simulink model "ReemcROStestlink"  (R2015a)
settings: Solver=ode45  StartTime=0.0  StopTime=inf  RelTol=1e-3
model workspace (MAT data in the model file):
  SL_ROS_VariableLengthArrays_MaxSizes.CommonInfo.ArrayTruncateAction = 'EmitWarning'
  SL_ROS_VariableLengthArrays_MaxSizes.MsgTypeMap = containers.Map
  SL_ROS_VariableLengthArrays_MaxSizes.MsgTypeMap.serialization.keys = {'gazebo_msgs/LinkStates'}
  SL_ROS_VariableLengthArrays_MaxSizes.MsgTypeMap.serialization.values{1}(1).PropertyName = 'Pose'
  SL_ROS_VariableLengthArrays_MaxSizes.MsgTypeMap.serialization.values{1}(1).DataType = 'geometry_msgs/Pose'
  SL_ROS_VariableLengthArrays_MaxSizes.MsgTypeMap.serialization.values{1}(1).MaxLength = 60
  SL_ROS_VariableLengthArrays_MaxSizes.MsgTypeMap.serialization.values{1}(2).PropertyName = 'Twist'
  SL_ROS_VariableLengthArrays_MaxSizes.MsgTypeMap.serialization.values{1}(2).DataType = 'geometry_msgs/Twist'
  SL_ROS_VariableLengthArrays_MaxSizes.MsgTypeMap.serialization.values{1}(2).MaxLength = 60
  SL_ROS_VariableLengthArrays_MaxSizes.MsgTypeMap.serialization.uniformity = 0
  SL_ROS_VariableLengthArrays_MaxSizes.MsgTypeMap.serialization.keyType = 'char'
  SL_ROS_VariableLengthArrays_MaxSizes.MsgTypeMap.serialization.valueType = 'any'
values from neighbouring files (symbols this model uses):
  left_ft = struct('force',0,'torqueX',0,'torqueY',0)    [Feedback.m]
  right_ft = struct('force',0,'torqueX',0,'torqueY',0)    [Feedback.m]
libraries: robotlib x13
settings Model: Creator=jifeixu  LastModifiedBy=jifeixu
settings OptimizationCC: BlockReduction=off  BufferReuse=off
settings DebuggingCC: AlgebraicLoopMsg=none  UnconnectedInputMsg=none  UnconnectedOutputMsg=none  UnconnectedLineMsg=none

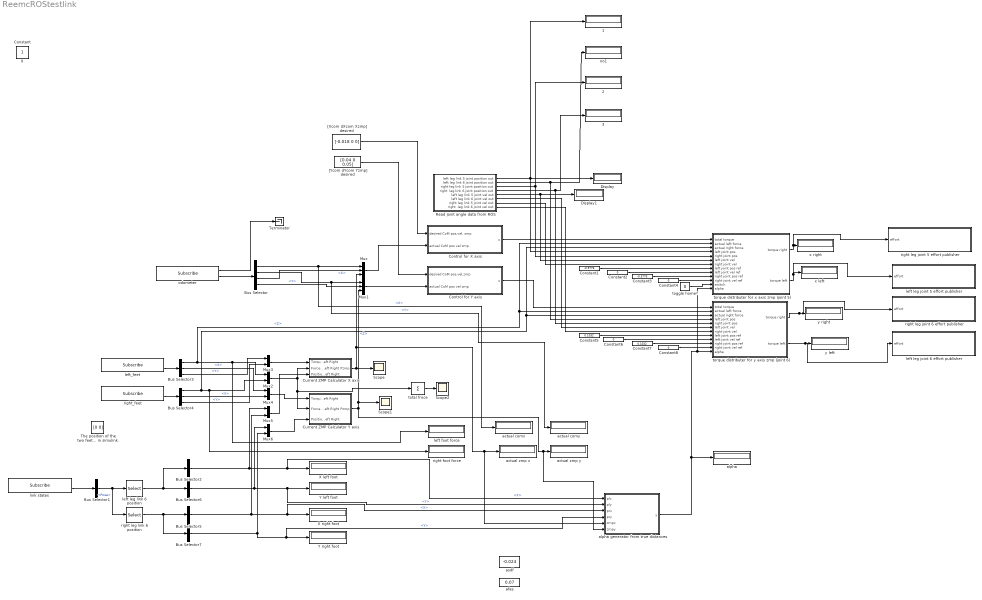
== system ReemcROStestlink ==
  1 : Display
  2 : Display
  3 : Display
  Bus Selector : BusSelector  OutputSignals=Pose.Pose.Position.X,Pose.Pose.Position.Y,Twist.Twist.Linear.X,Twist.Twist.Linear.Y
  Bus Selector1 : BusSelector  OutputSignals=Pose
  Bus Selector2 : BusSelector  OutputSignals=Position.X
  Bus Selector3 : BusSelector  OutputSignals=Wrench.Force.Z,Wrench.Torque.X,Wrench.Torque.Y
  Bus Selector4 : BusSelector  OutputSignals=Wrench.Force.Z,Wrench.Torque.X,Wrench.Torque.Y
  Bus Selector5 : BusSelector  OutputSignals=Position.X
  Bus Selector6 : BusSelector  OutputSignals=Position.Y
  Bus Selector7 : BusSelector  OutputSignals=Position.Y
  Constant1 : Constant  Value=-0.5776
  Constant{2,4,6,8} (4 alike) : Constant  Value=0
  Constant3 : Constant  Value=-0.5776
  Constant5 : Constant  Value=0.1032
  Constant7 : Constant  Value=0.1032
  Control for X axis : Subsystem
  Control for Y axis : Subsystem
  Current ZMP Calculator X axis : Subsystem
  Current ZMP Calculator Y axis : Subsystem
  Display : Display
  Display1 : Display
  Mux : Mux  Inputs=3
  Mux1 : Mux  Inputs=3
  Mux{2..6} (5 alike) : Mux  Inputs=2
  Read joint angle data from ROS : Subsystem
  Scope : Scope
      settings: YMin=-0.08  YMax=0.14
  Scope1 : Scope
      settings: YMin=-0.225  YMax=0.05
  Scope2 : Scope
      settings: YMin=-100  YMax=1700  SaveName=ScopeData2
  Terminator : Terminator
  The position of the two feet that should have come from the link state subscriber but currently does not work in simulink. : Constant  Value=[0 0]
  X left foot : Display
  X right foot : Display
  Y left foot : Display
  Y right foot : Display
  "[Xcom dXcom Xzmp] desired" : Constant  Value=[-0.018 0 0]  VectorParams1D=off
  "[Ycom dYcom Yzmp] desired" : Constant  Value=[0.04 0 0.05]  VectorParams1D=off
  actual comx : Display
  actual comy : Display
  actual zmp x : Display
  actual zmp y : Display
  afas : Constant  Value=0.07
  alpha : Display
  alpha generator from true distances : MATLAB Function  TreatAsAtomicUnit=on
  asdf : Constant  Value=-0.024
  left foot force : Display
  left leg joint 5 effort publisher : Subsystem
  left leg joint 6 effort publisher : Subsystem
  left leg link 6 position : Selector  InputPortWidth=60  Indices=8  OutputSizes=2
  left_feet : robotlib/Subscribe  SourceLibraryInfo=This block requires Robotics System Toolbox  topicSource=Select from ROS network  topic=/left_ft  messageType=geometry_msgs/WrenchStamped  sampleTime=-1  messageQueueLength=1
  link states : robotlib/Subscribe  SourceLibraryInfo=This block requires Robotics System Toolbox  topicSource=Select from ROS network  topic=/gazebo/link_states  messageType=gazebo_msgs/LinkStates  sampleTime=-1  messageQueueLength=1
  no1 : Display
  odometer : robotlib/Subscribe  SourceLibraryInfo=This block requires Robotics System Toolbox  topicSource=Select from ROS network  topic=/ground_truth_odom  messageType=nav_msgs/Odometry  sampleTime=-1  messageQueueLength=1
  right foot force : Display
  right leg joint 5 effort publisher : Subsystem
  right leg joint 6 effort publisher : Subsystem
  right leg link 6 position : Selector  InputPortWidth=60  Indices=14  OutputSizes=2
  right_feet : robotlib/Subscribe  SourceLibraryInfo=This block requires Robotics System Toolbox  topicSource=Select from ROS network  topic=/right_ft  messageType=geometry_msgs/WrenchStamped  sampleTime=-1  messageQueueLength=1
  toggle home? : Constant  Value=0
  torque distributer for x axis zmp (joint 5) : Subsystem
  torque distributer for y axis zmp (joint 6) : Subsystem
  total froce : Sum  Inputs=+
  x left : Display
  x right : Display
  y left : Display
  y right : Display
  0 : Constant  IOType=siggen
  Constant : Constant  IOType=siggen
  wires:
  odometer/2 -> Bus Selector/1
  odometer/1 -> Terminator/1
  left_feet/2 -> Bus Selector3/1
  right_feet/2 -> Bus Selector4/1
  Bus Selector/1 -> actual comx/1, Mux/1  "<X>"
  Bus Selector/3 -> Mux/2  "<X>"
  Bus Selector/2 -> actual comy/1, Mux1/1  "<Y>"
  Bus Selector/4 -> Mux1/2  "<Y>"
  Current ZMP Calculator X axis/1(Pzmp) -> Scope/1, alpha generator from true distances/5(zmpx), actual zmp x/1, Mux/3
  Current ZMP Calculator Y axis/1(Pzmp) -> Mux1/3, Scope1/1, alpha generator from true distances/6(zmpy), actual zmp y/1
  "[Xcom dXcom Xzmp] desired"/1 -> Control for X axis/1("desired CoM pos,vel, zmp")
  Mux/1 -> Control for X axis/2("actual CoM pos vel zmp ")
  Mux2/1 -> total froce/1, Current ZMP Calculator Y axis/2(Force Left Right), Current ZMP Calculator X axis/2(Force Left Right)
  Bus Selector3/1 -> torque distributer for y axis zmp (joint 6)/2(actual left force), torque distributer for x axis zmp (joint 5)/2(actual left force), left foot force/1, Mux2/1  "<Z>"
  Bus Selector4/1 -> torque distributer for y axis zmp (joint 6)/3(actual right force), torque distributer for x axis zmp (joint 5)/3(actual right force), right foot force/1, Mux2/2  "<Z>"
  Mux3/1 -> Current ZMP Calculator X axis/1(Torque Left Right)
  Mux4/1 -> Current ZMP Calculator Y axis/1(Torque Left Right)
  Bus Selector3/3 -> Mux3/1  "<Y>"
  Bus Selector4/3 -> Mux3/2  "<Y>"
  Bus Selector3/2 -> Mux4/1  "<X>"
  Bus Selector4/2 -> Mux4/2  "<X>"
  Mux1/1 -> Control for Y axis/2("actual CoM pos vel zmp ")
  "[Ycom dYcom Yzmp] desired"/1 -> Control for Y axis/1(desired CoM pos,vel,zmp)
  link states/2 -> Bus Selector1/1
  Bus Selector1/1 -> right leg link 6 position/1, left leg link 6 position/1  "<Pose>"
  Bus Selector2/1 -> Mux5/1, alpha generator from true distances/1(plx), X left foot/1  "<X>"
  Control for X axis/1(u) -> torque distributer for x axis zmp (joint 5)/1(total torque)
  left leg link 6 position/1 -> Bus Selector2/1, Bus Selector6/1
  Bus Selector5/1 -> Mux5/2, alpha generator from true distances/3(prx), X right foot/1  "<X>"
  right leg link 6 position/1 -> Bus Selector7/1, Bus Selector5/1
  Bus Selector6/1 -> Mux6/1, alpha generator from true distances/2(ply), Y left foot/1  "<Y>"
  Bus Selector7/1 -> alpha generator from true distances/4(pry), Y right foot/1, Mux6/2  "<Y>"
  Mux5/1 -> Current ZMP Calculator X axis/3(Position Left Right)
  Mux6/1 -> Current ZMP Calculator Y axis/3(Position Left Right)
  total froce/1 -> Scope2/1
  Read joint angle data from ROS/1(left leg link 5 joint position out) -> Display/1, 1/1, torque distributer for x axis zmp (joint 5)/4(left joint pos)
  Read joint angle data from ROS/3(right leg link 5 joint position out) -> torque distributer for x axis zmp (joint 5)/5(right joint pos), 2/1
  Read joint angle data from ROS/2(left leg link 6 joint position out) -> torque distributer for y axis zmp (joint 6)/4(left joint pos), no1/1
  Read joint angle data from ROS/4(right  leg link 6 joint position out) -> torque distributer for y axis zmp (joint 6)/5(right joint pos), 3/1
  Read joint angle data from ROS/5(left leg link 5 joint vel out) -> Display1/1, torque distributer for x axis zmp (joint 5)/6(left joint vel)
  Read joint angle data from ROS/7(right leg link 5 joint vel out) -> torque distributer for x axis zmp (joint 5)/7(right joint vel)
  torque distributer for x axis zmp (joint 5)/1(torque right) -> right leg joint 5 effort publisher/1(effort), x right/1
  torque distributer for x axis zmp (joint 5)/2(torque left) -> x left/1, left leg joint 5 effort publisher/1(effort)
  Read joint angle data from ROS/6(left leg link 6 joint vel out) -> torque distributer for y axis zmp (joint 6)/6(left joint vel)
  Read joint angle data from ROS/8(right  leg link 6 joint vel out) -> torque distributer for y axis zmp (joint 6)/7(right joint vel)
  torque distributer for y axis zmp (joint 6)/1(torque right) -> right leg joint 6 effort publisher/1(effort), y right/1
  Control for Y axis/1(u) -> torque distributer for y axis zmp (joint 6)/1(total torque)
  Constant1/1 -> torque distributer for x axis zmp (joint 5)/8(left joint pos ref)
  Constant2/1 -> torque distributer for x axis zmp (joint 5)/9(left joint vel ref)
  Constant3/1 -> torque distributer for x axis zmp (joint 5)/10(right joint pos ref)
  Constant4/1 -> torque distributer for x axis zmp (joint 5)/11(right joint vel ref)
  Constant5/1 -> torque distributer for y axis zmp (joint 6)/8(left joint pos ref)
  Constant6/1 -> torque distributer for y axis zmp (joint 6)/9(left joint vel ref)
  Constant7/1 -> torque distributer for y axis zmp (joint 6)/10(right joint pos ref)
  Constant8/1 -> torque distributer for y axis zmp (joint 6)/11(right joint vel ref)
  torque distributer for y axis zmp (joint 6)/2(torque left) -> left leg joint 6 effort publisher/1(effort), y left/1
  toggle home?/1 -> torque distributer for x axis zmp (joint 5)/12(switch)
  alpha generator from true distances/1(y) -> alpha/1, torque distributer for x axis zmp (joint 5)/13(alpha), torque distributer for y axis zmp (joint 6)/12(alpha)

== system ReemcROStestlink/Control for X axis ==
  "desired CoM pos,vel, zmp" : Inport
  "actual CoM pos vel zmp " : Inport  Port=2
  Add : Sum
  Demux : Demux  Outputs=3
  K gains : Constant  Value="[ -3235   -150    20.5]"  VectorParams1D=off
  Permute Dimensions : PermuteDimensions
  Product : Product  Multiplication=Matrix(*)
  Subtract : Sum  Inputs=+-
  u : Outport
  wires:
  "desired CoM pos,vel, zmp"/1 -> Demux/1, Subtract/1
  K gains/1 -> Product/1
  Subtract/1 -> Permute Dimensions/1
  "actual CoM pos vel zmp "/1 -> Subtract/2
  Product/1 -> Add/2
  Add/1 -> u/1
  Demux/3 -> Add/1
  Permute Dimensions/1 -> Product/2

== system ReemcROStestlink/Control for Y axis ==
  desired CoM pos,vel,zmp : Inport
  "actual CoM pos vel zmp " : Inport  Port=2
  Add : Sum
  Demux : Demux  Outputs=3
  K gains : Constant  Value="[ -3235   -150    20.5]"  VectorParams1D=off
  Permute Dimensions : PermuteDimensions
  Product : Product  Multiplication=Matrix(*)
  Subtract : Sum  Inputs=+-
  u : Outport
  wires:
  K gains/1 -> Product/1
  "actual CoM pos vel zmp "/1 -> Subtract/2
  Product/1 -> Add/2
  Add/1 -> u/1
  Permute Dimensions/1 -> Product/2
  Subtract/1 -> Permute Dimensions/1
  desired CoM pos,vel,zmp/1 -> Demux/1, Subtract/1
  Demux/3 -> Add/1

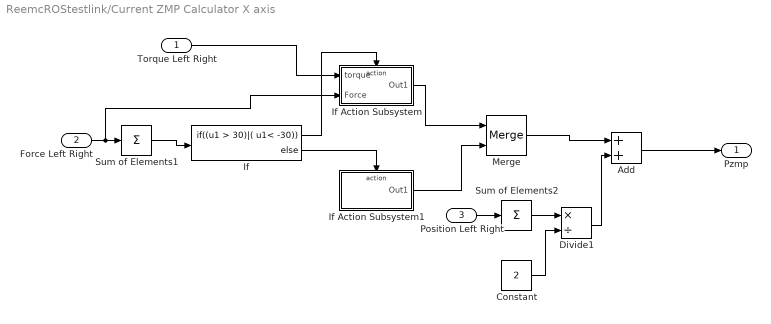
== system ReemcROStestlink/Current ZMP Calculator X axis ==
  Torque Left Right : Inport
  Force Left Right : Inport  Port=2
  Position Left Right : Inport  Port=3
  Add : Sum
  Constant : Constant  Value=2
  Divide1 : Product  Inputs=*/
  If : If  IfExpression=(u1 > 30)|( u1< -30)
  If Action Subsystem : Subsystem  TreatAsAtomicUnit=on
  If Action Subsystem1 : Subsystem  TreatAsAtomicUnit=on
  Merge : Merge
  Sum of Elements1 : Sum  Inputs=+
  Sum of Elements2 : Sum  Inputs=+
  Pzmp : Outport
  wires:
  Force Left Right/1 -> If Action Subsystem/2(Force), Sum of Elements1/1
  Sum of Elements1/1 -> If/1
  If Action Subsystem1/1(Out1) -> Merge/2
  Merge/1 -> Add/1
  Add/1 -> Pzmp/1
  Position Left Right/1 -> Sum of Elements2/1
  Sum of Elements2/1 -> Divide1/1
  Constant/1 -> Divide1/2
  Divide1/1 -> Add/2
  Torque Left Right/1 -> If Action Subsystem/1(torque)
  If Action Subsystem/1(Out1) -> Merge/1
  If/1 -> If Action Subsystem/Action
  If/2 -> If Action Subsystem1/Action

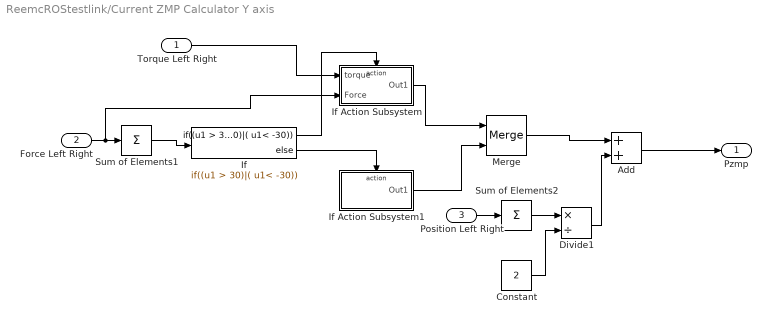
== system ReemcROStestlink/Current ZMP Calculator Y axis ==
  Torque Left Right : Inport
  Force Left Right : Inport  Port=2
  Position Left Right : Inport  Port=3
  Add : Sum
  Constant : Constant  Value=2
  Divide1 : Product  Inputs=*/
  If : If  IfExpression=(u1 > 30)|( u1< -30)
  If Action Subsystem : Subsystem  TreatAsAtomicUnit=on
  If Action Subsystem1 : Subsystem  TreatAsAtomicUnit=on
  Merge : Merge
  Sum of Elements1 : Sum  Inputs=+
  Sum of Elements2 : Sum  Inputs=+
  Pzmp : Outport
  wires:
  Force Left Right/1 -> If Action Subsystem/2(Force), Sum of Elements1/1
  Sum of Elements1/1 -> If/1
  If Action Subsystem1/1(Out1) -> Merge/2
  Merge/1 -> Add/1
  Add/1 -> Pzmp/1
  Position Left Right/1 -> Sum of Elements2/1
  Sum of Elements2/1 -> Divide1/1
  Constant/1 -> Divide1/2
  Divide1/1 -> Add/2
  Torque Left Right/1 -> If Action Subsystem/1(torque)
  If Action Subsystem/1(Out1) -> Merge/1
  If/1 -> If Action Subsystem/Action
  If/2 -> If Action Subsystem1/Action

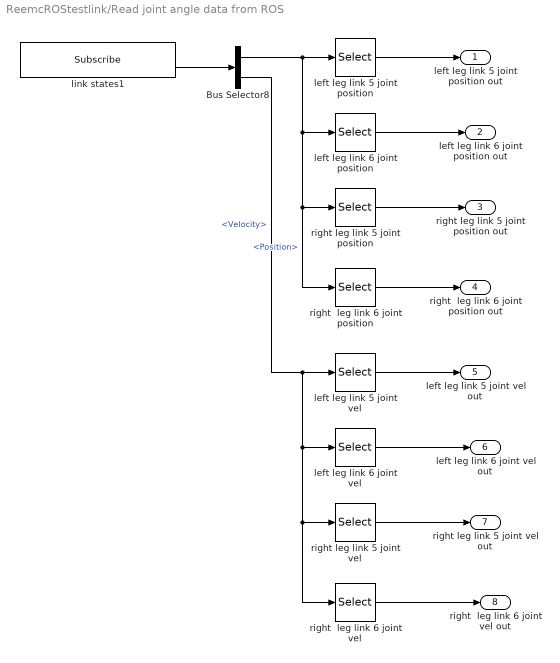
== system ReemcROStestlink/Read joint angle data from ROS ==
  Bus Selector8 : BusSelector  OutputSignals=Position,Velocity
  left leg link 5 joint position : Selector  InputPortWidth=128  Indices=39  OutputSizes=2
  left leg link 5 joint vel : Selector  InputPortWidth=128  Indices=39  OutputSizes=2
  left leg link 6 joint position : Selector  InputPortWidth=128  Indices=40  OutputSizes=2
  left leg link 6 joint vel : Selector  InputPortWidth=128  Indices=40  OutputSizes=2
  link states1 : robotlib/Subscribe  SourceLibraryInfo=This block requires Robotics System Toolbox  topicSource=Select from ROS network  topic=/joint_states  messageType=sensor_msgs/JointState  sampleTime=-1  messageQueueLength=1
  right  leg link 6 joint position : Selector  InputPortWidth=128  Indices=46  OutputSizes=2
  right  leg link 6 joint vel : Selector  InputPortWidth=128  Indices=46  OutputSizes=2
  right leg link 5 joint position : Selector  InputPortWidth=128  Indices=45  OutputSizes=2
  right leg link 5 joint vel : Selector  InputPortWidth=128  Indices=45  OutputSizes=2
  left leg link 5 joint position out : Outport
  left leg link 6 joint position out : Outport  Port=2
  right leg link 5 joint position out : Outport  Port=3
  right  leg link 6 joint position out : Outport  Port=4
  left leg link 5 joint vel out : Outport  Port=5
  left leg link 6 joint vel out : Outport  Port=6
  right leg link 5 joint vel out : Outport  Port=7
  right  leg link 6 joint vel out : Outport  Port=8
  wires:
  Bus Selector8/1 -> left leg link 6 joint position/1, right  leg link 6 joint position/1, right leg link 5 joint position/1, left leg link 5 joint position/1  "<Position>"
  left leg link 5 joint position/1 -> left leg link 5 joint position out/1
  left leg link 6 joint position/1 -> left leg link 6 joint position out/1
  link states1/2 -> Bus Selector8/1
  right leg link 5 joint position/1 -> right leg link 5 joint position out/1
  right  leg link 6 joint position/1 -> right  leg link 6 joint position out/1
  Bus Selector8/2 -> left leg link 6 joint vel/1, right  leg link 6 joint vel/1, right leg link 5 joint vel/1, left leg link 5 joint vel/1  "<Velocity>"
  left leg link 5 joint vel/1 -> left leg link 5 joint vel out/1
  left leg link 6 joint vel/1 -> left leg link 6 joint vel out/1
  right leg link 5 joint vel/1 -> right leg link 5 joint vel out/1
  right  leg link 6 joint vel/1 -> right  leg link 6 joint vel out/1

== system ReemcROStestlink/left leg joint 5 effort publisher ==
  effort : Inport
  Blank Message : robotlib/Blank Message  SourceLibraryInfo=This block requires Robotics System Toolbox  messageType=std_msgs/Float64  SampleTime=inf
  Bus Assignment : BusAssignment  AssignedSignals=Data
  Publish : robotlib/Publish  SourceLibraryInfo=This block requires Robotics System Toolbox  topicSource=Select from ROS network  topic=/left_leg_effort_controller2/command  messageType=std_msgs/Float64  messageQueueLength=1
  wires:
  effort/1 -> Bus Assignment/2
  Bus Assignment/1 -> Publish/1
  Blank Message/1 -> Bus Assignment/1

== system ReemcROStestlink/left leg joint 6 effort publisher ==
  effort : Inport
  Blank Message : robotlib/Blank Message  SourceLibraryInfo=This block requires Robotics System Toolbox  messageType=std_msgs/Float64  SampleTime=inf
  Bus Assignment : BusAssignment  AssignedSignals=Data
  Publish : robotlib/Publish  SourceLibraryInfo=This block requires Robotics System Toolbox  topicSource=Select from ROS network  topic=/left_leg_effort_controller3/command  messageType=std_msgs/Float64  messageQueueLength=1
  wires:
  effort/1 -> Bus Assignment/2
  Bus Assignment/1 -> Publish/1
  Blank Message/1 -> Bus Assignment/1

== system ReemcROStestlink/right leg joint 5 effort publisher ==
  effort : Inport
  Blank Message : robotlib/Blank Message  SourceLibraryInfo=This block requires Robotics System Toolbox  messageType=std_msgs/Float64  SampleTime=inf
  Bus Assignment : BusAssignment  AssignedSignals=Data
  Publish2 : robotlib/Publish  SourceLibraryInfo=This block requires Robotics System Toolbox  topicSource=Select from ROS network  topic=/right_leg_effort_controller2/command  messageType=std_msgs/Float64  messageQueueLength=1
  wires:
  effort/1 -> Bus Assignment/2
  Bus Assignment/1 -> Publish2/1
  Blank Message/1 -> Bus Assignment/1

== system ReemcROStestlink/right leg joint 6 effort publisher ==
  effort : Inport
  Blank Message : robotlib/Blank Message  SourceLibraryInfo=This block requires Robotics System Toolbox  messageType=std_msgs/Float64  SampleTime=inf
  Bus Assignment : BusAssignment  AssignedSignals=Data
  Publish2 : robotlib/Publish  SourceLibraryInfo=This block requires Robotics System Toolbox  topicSource=Select from ROS network  topic=/right_leg_effort_controller3/command  messageType=std_msgs/Float64  messageQueueLength=1
  wires:
  effort/1 -> Bus Assignment/2
  Bus Assignment/1 -> Publish2/1
  Blank Message/1 -> Bus Assignment/1

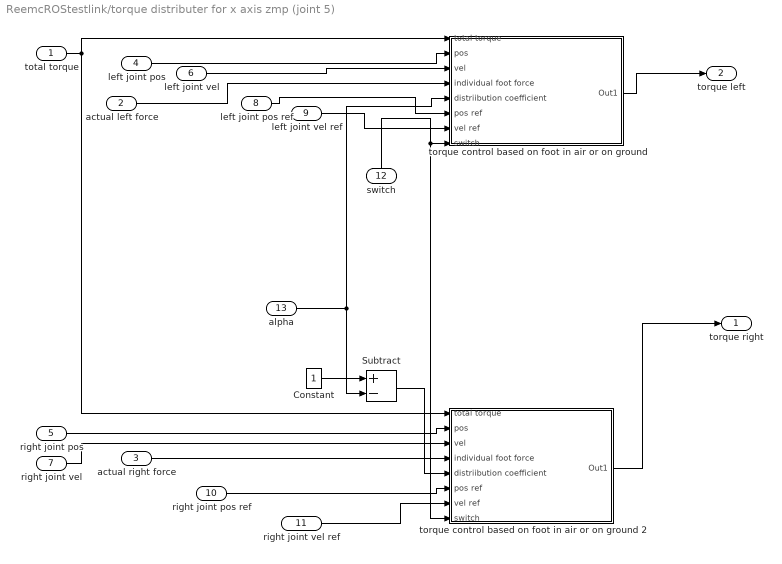
== system ReemcROStestlink/torque distributer for x axis zmp (joint 5) ==
  total torque : Inport
  actual left force : Inport  Port=2
  actual right force : Inport  Port=3
  left joint pos : Inport  Port=4
  right joint pos : Inport  Port=5
  left joint vel : Inport  Port=6
  right joint vel : Inport  Port=7
  left joint pos ref : Inport  Port=8
  left joint vel ref : Inport  Port=9
  right joint pos ref : Inport  Port=10
  right joint vel ref : Inport  Port=11
  switch : Inport  Port=12
  alpha : Inport  Port=13
  Constant : Constant
  Subtract : Sum  Inputs=+-
  torque control based on foot in air or on ground : Subsystem
  torque control based on foot in air or on ground 2 : Subsystem
  torque right : Outport
  torque left : Outport  Port=2
  wires:
  total torque/1 -> torque control based on foot in air or on ground 2/1(total torque), torque control based on foot in air or on ground/1(total torque)
  left joint pos/1 -> torque control based on foot in air or on ground/2(pos)
  left joint vel/1 -> torque control based on foot in air or on ground/3(vel)
  alpha/1 -> Subtract/2, torque control based on foot in air or on ground/5(distriibution coefficient)
  torque control based on foot in air or on ground/1(Out1) -> torque left/1
  right joint pos/1 -> torque control based on foot in air or on ground 2/2(pos)
  right joint vel/1 -> torque control based on foot in air or on ground 2/3(vel)
  Constant/1 -> Subtract/1
  Subtract/1 -> torque control based on foot in air or on ground 2/5(distriibution coefficient)
  torque control based on foot in air or on ground 2/1(Out1) -> torque right/1
  left joint pos ref/1 -> torque control based on foot in air or on ground/6(pos ref)
  left joint vel ref/1 -> torque control based on foot in air or on ground/7(vel ref)
  right joint pos ref/1 -> torque control based on foot in air or on ground 2/6(pos ref)
  right joint vel ref/1 -> torque control based on foot in air or on ground 2/7(vel ref)
  switch/1 -> torque control based on foot in air or on ground 2/8(switch), torque control based on foot in air or on ground/8(switch)
  actual right force/1 -> torque control based on foot in air or on ground 2/4(individual foot force)
  actual left force/1 -> torque control based on foot in air or on ground/4(individual foot force)

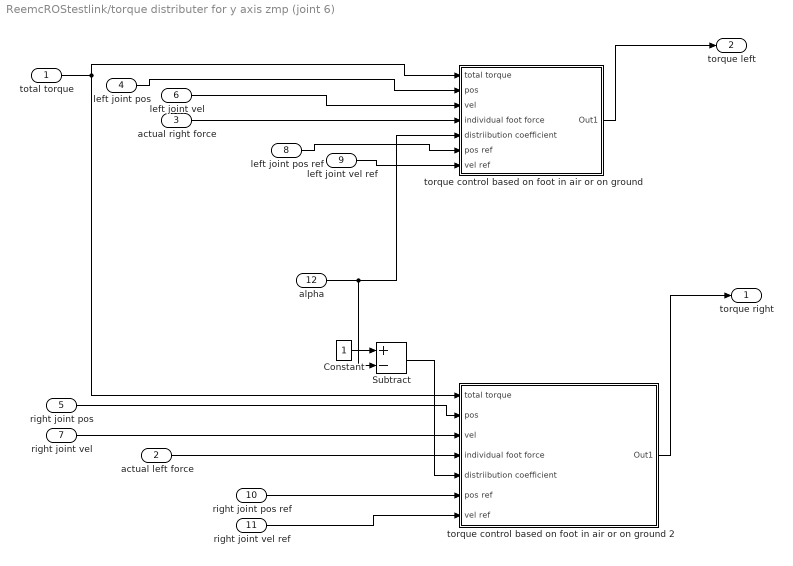
== system ReemcROStestlink/torque distributer for y axis zmp (joint 6) ==
  total torque : Inport
  actual left force : Inport  Port=2
  actual right force : Inport  Port=3
  left joint pos : Inport  Port=4
  right joint pos : Inport  Port=5
  left joint vel : Inport  Port=6
  right joint vel : Inport  Port=7
  left joint pos ref : Inport  Port=8
  left joint vel ref : Inport  Port=9
  right joint pos ref : Inport  Port=10
  right joint vel ref : Inport  Port=11
  alpha : Inport  Port=12
  Constant : Constant
  Subtract : Sum  Inputs=+-
  torque control based on foot in air or on ground : Subsystem
  torque control based on foot in air or on ground 2 : Subsystem
  torque right : Outport
  torque left : Outport  Port=2
  wires:
  actual left force/1 -> torque control based on foot in air or on ground 2/4(individual foot force)
  actual right force/1 -> torque control based on foot in air or on ground/4(individual foot force)
  total torque/1 -> torque control based on foot in air or on ground/1(total torque), torque control based on foot in air or on ground 2/1(total torque)
  left joint pos/1 -> torque control based on foot in air or on ground/2(pos)
  left joint vel/1 -> torque control based on foot in air or on ground/3(vel)
  alpha/1 -> torque control based on foot in air or on ground/5(distriibution coefficient), Subtract/2
  torque control based on foot in air or on ground/1(Out1) -> torque left/1
  right joint pos/1 -> torque control based on foot in air or on ground 2/2(pos)
  right joint vel/1 -> torque control based on foot in air or on ground 2/3(vel)
  Constant/1 -> Subtract/1
  Subtract/1 -> torque control based on foot in air or on ground 2/5(distriibution coefficient)
  torque control based on foot in air or on ground 2/1(Out1) -> torque right/1
  left joint pos ref/1 -> torque control based on foot in air or on ground/6(pos ref)
  left joint vel ref/1 -> torque control based on foot in air or on ground/7(vel ref)
  right joint vel ref/1 -> torque control based on foot in air or on ground 2/7(vel ref)
  right joint pos ref/1 -> torque control based on foot in air or on ground 2/6(pos ref)

== system ReemcROStestlink/Current ZMP Calculator X axis/If Action Subsystem ==
  torque : Inport
  Force : Inport  Port=2
  Action Port : ActionPort  ActionType=then
  Divide : Product  Inputs=*/
  Gain : Gain  Gain=-1
  Sum of Elements : Sum  Inputs=+
  Sum of Elements1 : Sum  Inputs=+
  Out1 : Outport
  wires:
  Divide/1 -> Out1/1
  Gain/1 -> Divide/1
  torque/1 -> Sum of Elements/1
  Sum of Elements/1 -> Gain/1
  Force/1 -> Sum of Elements1/1
  Sum of Elements1/1 -> Divide/2

== system ReemcROStestlink/Current ZMP Calculator X axis/If Action Subsystem1 ==
  Action Port : ActionPort  ActionType=else
  Constant1 : Constant  Value=0
  Out1 : Outport
  wires:
  Constant1/1 -> Out1/1

== system ReemcROStestlink/Current ZMP Calculator Y axis/If Action Subsystem ==
  torque : Inport
  Force : Inport  Port=2
  Action Port : ActionPort  ActionType=then
  Divide : Product  Inputs=*/
  Gain : Gain  Gain=-1
  Sum of Elements : Sum  Inputs=+
  Sum of Elements1 : Sum  Inputs=+
  Out1 : Outport
  wires:
  Divide/1 -> Out1/1
  Gain/1 -> Divide/1
  torque/1 -> Sum of Elements/1
  Sum of Elements/1 -> Gain/1
  Force/1 -> Sum of Elements1/1
  Sum of Elements1/1 -> Divide/2

== system ReemcROStestlink/Current ZMP Calculator Y axis/If Action Subsystem1 ==
  Action Port : ActionPort  ActionType=else
  Constant1 : Constant  Value=0
  Out1 : Outport
  wires:
  Constant1/1 -> Out1/1

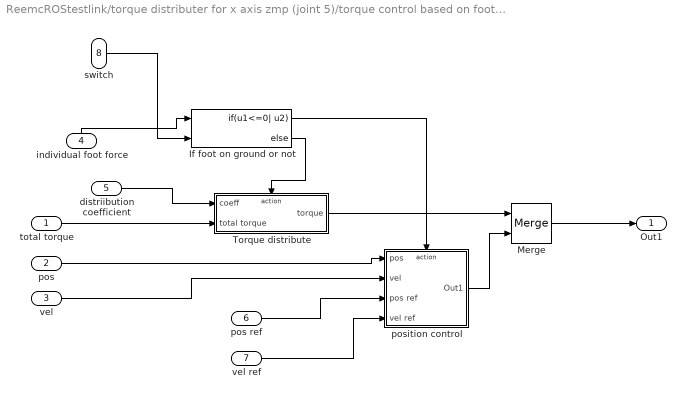
== system ReemcROStestlink/torque distributer for x axis zmp (joint 5)/torque control based on foot in air or on ground ==
  total torque : Inport
  pos : Inport  Port=2
  vel : Inport  Port=3
  individual foot force : Inport  Port=4
  distriibution coefficient : Inport  Port=5
  pos ref : Inport  Port=6
  vel ref : Inport  Port=7
  switch : Inport  Port=8
  If foot on ground or not : If  NumInputs=2  IfExpression=u1<=0| u2
  Merge : Merge
  Torque distribute : Subsystem  TreatAsAtomicUnit=on
  position control : Subsystem  TreatAsAtomicUnit=on
  Out1 : Outport
  wires:
  Merge/1 -> Out1/1
  If foot on ground or not/2 -> Torque distribute/Action
  If foot on ground or not/1 -> position control/Action
  pos/1 -> position control/1(pos)
  individual foot force/1 -> If foot on ground or not/1
  distriibution coefficient/1 -> Torque distribute/1(coeff)
  total torque/1 -> Torque distribute/2(total torque)
  position control/1(Out1) -> Merge/2
  Torque distribute/1(torque) -> Merge/1
  pos ref/1 -> position control/3(pos ref)
  vel ref/1 -> position control/4(vel ref)
  vel/1 -> position control/2(vel)
  switch/1 -> If foot on ground or not/2

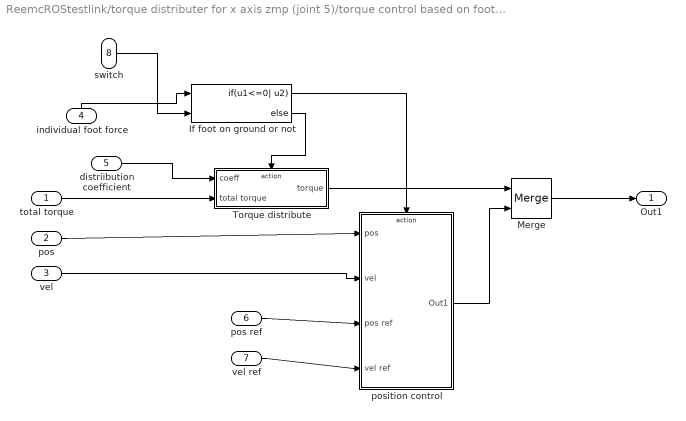
== system ReemcROStestlink/torque distributer for x axis zmp (joint 5)/torque control based on foot in air or on ground 2 ==
  total torque : Inport
  pos : Inport  Port=2
  vel : Inport  Port=3
  individual foot force : Inport  Port=4
  distriibution coefficient : Inport  Port=5
  pos ref : Inport  Port=6
  vel ref : Inport  Port=7
  switch : Inport  Port=8
  If foot on ground or not : If  NumInputs=2  IfExpression=u1<=0| u2
  Merge : Merge
  Torque distribute : Subsystem  TreatAsAtomicUnit=on
  position control : Subsystem  TreatAsAtomicUnit=on
  Out1 : Outport
  wires:
  Merge/1 -> Out1/1
  If foot on ground or not/2 -> Torque distribute/Action
  If foot on ground or not/1 -> position control/Action
  pos/1 -> position control/1(pos)
  individual foot force/1 -> If foot on ground or not/1
  distriibution coefficient/1 -> Torque distribute/1(coeff)
  total torque/1 -> Torque distribute/2(total torque)
  vel/1 -> position control/2(vel)
  position control/1(Out1) -> Merge/2
  Torque distribute/1(torque) -> Merge/1
  pos ref/1 -> position control/3(pos ref)
  vel ref/1 -> position control/4(vel ref)
  switch/1 -> If foot on ground or not/2

== system ReemcROStestlink/torque distributer for y axis zmp (joint 6)/torque control based on foot in air or on ground ==
  total torque : Inport
  pos : Inport  Port=2
  vel : Inport  Port=3
  individual foot force : Inport  Port=4
  distriibution coefficient : Inport  Port=5
  pos ref : Inport  Port=6
  vel ref : Inport  Port=7
  If foot on ground or not : If  IfExpression=u1<=10000
  Merge : Merge
  Torque distribute : Subsystem  TreatAsAtomicUnit=on
  position control : Subsystem  TreatAsAtomicUnit=on
  Out1 : Outport
  wires:
  Merge/1 -> Out1/1
  If foot on ground or not/2 -> Torque distribute/Action
  If foot on ground or not/1 -> position control/Action
  pos/1 -> position control/1(pos)
  individual foot force/1 -> If foot on ground or not/1
  distriibution coefficient/1 -> Torque distribute/1(coeff)
  total torque/1 -> Torque distribute/2(total torque)
  vel/1 -> position control/2(vel)
  position control/1(Out1) -> Merge/2
  Torque distribute/1(torque) -> Merge/1
  pos ref/1 -> position control/3(pos ref)
  vel ref/1 -> position control/4(vel ref)

== system ReemcROStestlink/torque distributer for y axis zmp (joint 6)/torque control based on foot in air or on ground 2 ==
  total torque : Inport
  pos : Inport  Port=2
  vel : Inport  Port=3
  individual foot force : Inport  Port=4
  distriibution coefficient : Inport  Port=5
  pos ref : Inport  Port=6
  vel ref : Inport  Port=7
  If foot on ground or not : If  IfExpression=u1<=10000
  Merge : Merge
  Torque distribute : Subsystem  TreatAsAtomicUnit=on
  position control : Subsystem  TreatAsAtomicUnit=on
  Out1 : Outport
  wires:
  Merge/1 -> Out1/1
  If foot on ground or not/2 -> Torque distribute/Action
  If foot on ground or not/1 -> position control/Action
  pos/1 -> position control/1(pos)
  individual foot force/1 -> If foot on ground or not/1
  distriibution coefficient/1 -> Torque distribute/1(coeff)
  total torque/1 -> Torque distribute/2(total torque)
  vel/1 -> position control/2(vel)
  position control/1(Out1) -> Merge/2
  Torque distribute/1(torque) -> Merge/1
  pos ref/1 -> position control/3(pos ref)
  vel ref/1 -> position control/4(vel ref)

== system ReemcROStestlink/torque distributer for x axis zmp (joint 5)/torque control based on foot in air or on ground/Torque distribute ==
  coeff : Inport
  total torque : Inport  Port=2
  Action Port : ActionPort  ActionType=else
  Gain : Gain
  Product : Product
  torque : Outport
  wires:
  coeff/1 -> Product/1
  total torque/1 -> Product/2
  Product/1 -> Gain/1
  Gain/1 -> torque/1

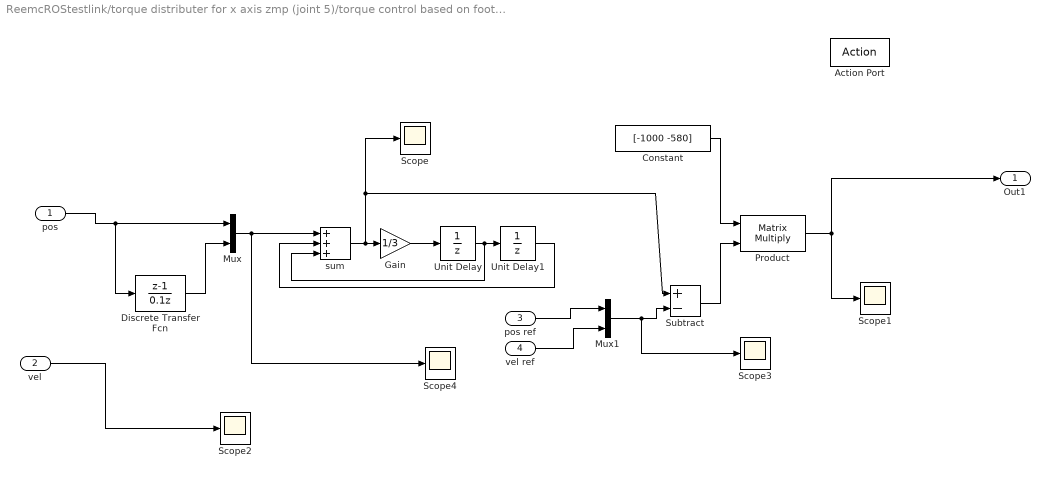
== system ReemcROStestlink/torque distributer for x axis zmp (joint 5)/torque control based on foot in air or on ground/position control ==
  pos : Inport
  vel : Inport  Port=2
  pos ref : Inport  Port=3
  vel ref : Inport  Port=4
  Action Port : ActionPort  ActionType=then
  Constant : Constant  Value=[-1000 -580]  VectorParams1D=off
  Discrete Transfer Fcn : DiscreteTransferFcn  Numerator=[1 -1]  Denominator=[0.1 0]  SampleTime=0.1
  Gain : Gain  Gain=1/3
  Mux : Mux  Inputs=[1;1]
  Mux1 : Mux  Inputs=[1;1]
  Product : Product  Multiplication=Matrix(*)
  Scope{,1..4} (5 alike) : Scope
      Scope settings: TimeRange=1.02  YMin=-18  YMax=2  SaveName=ScopeData5
      Scope1 settings: YMin=-6000  YMax=1500  SaveName=ScopeData6
      Scope2 settings: YMin=-8  YMax=15  SaveName=ScopeData11
      Scope3 settings: YMin=-0.6  YMax=0  SaveName=ScopeData12
      Scope4 settings: TimeRange=1.02  YMin=-18  YMax=1  SaveName=ScopeData13
  Subtract : Sum  Inputs=+-
  Unit Delay : UnitDelay  SampleTime=-1
  Unit Delay1 : UnitDelay  SampleTime=-1
  sum : Sum  Inputs=+++
  Out1 : Outport
  wires:
  pos/1 -> Discrete Transfer Fcn/1, Mux/1
  Constant/1 -> Product/1
  vel ref/1 -> Mux1/2
  pos ref/1 -> Mux1/1
  Mux1/1 -> Scope3/1, Subtract/2
  Subtract/1 -> Product/2
  sum/1 -> Scope/1, Subtract/1, Gain/1
  Gain/1 -> Unit Delay/1
  Unit Delay/1 -> sum/3, Unit Delay1/1
  Unit Delay1/1 -> sum/2
  vel/1 -> Scope2/1
  Discrete Transfer Fcn/1 -> Mux/2
  Product/1 -> Out1/1, Scope1/1
  Mux/1 -> Scope4/1, sum/1

== system ReemcROStestlink/torque distributer for x axis zmp (joint 5)/torque control based on foot in air or on ground 2/Torque distribute ==
  coeff : Inport
  total torque : Inport  Port=2
  Action Port : ActionPort  ActionType=else
  Gain : Gain
  Product : Product
  torque : Outport
  wires:
  coeff/1 -> Product/1
  total torque/1 -> Product/2
  Product/1 -> Gain/1
  Gain/1 -> torque/1

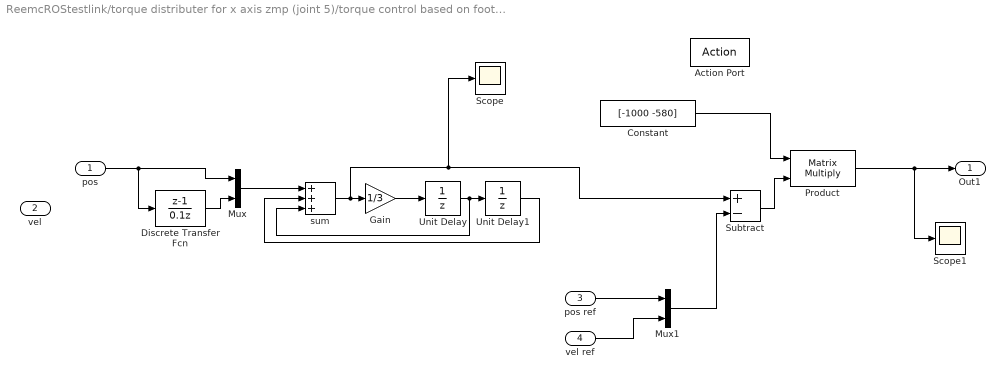
== system ReemcROStestlink/torque distributer for x axis zmp (joint 5)/torque control based on foot in air or on ground 2/position control ==
  pos : Inport
  vel : Inport  Port=2
  pos ref : Inport  Port=3
  vel ref : Inport  Port=4
  Action Port : ActionPort  ActionType=then
  Constant : Constant  Value=[-1000 -580]  VectorParams1D=off
  Discrete Transfer Fcn : DiscreteTransferFcn  Numerator=[1 -1]  Denominator=[0.1 0]  SampleTime=0.1
  Gain : Gain  Gain=1/3
  Mux : Mux  Inputs=[1;1]
  Mux1 : Mux  Inputs=[1;1]
  Product : Product  Multiplication=Matrix(*)
  Scope : Scope
      settings: YMin=-12.5  YMax=35  SaveName=ScopeData3
  Scope1 : Scope
      settings: YMin=-150  YMax=500  SaveName=ScopeData4
  Subtract : Sum  Inputs=+-
  Unit Delay : UnitDelay  SampleTime=-1
  Unit Delay1 : UnitDelay  SampleTime=-1
  sum : Sum  Inputs=+++
  Out1 : Outport
  wires:
  pos/1 -> Discrete Transfer Fcn/1, Mux/1
  Constant/1 -> Product/1
  vel ref/1 -> Mux1/2
  pos ref/1 -> Mux1/1
  Mux1/1 -> Subtract/2
  Subtract/1 -> Product/2
  Mux/1 -> sum/1
  sum/1 -> Scope/1, Subtract/1, Gain/1
  Gain/1 -> Unit Delay/1
  Unit Delay/1 -> sum/3, Unit Delay1/1
  Unit Delay1/1 -> sum/2
  Product/1 -> Scope1/1, Out1/1
  Discrete Transfer Fcn/1 -> Mux/2

== system ReemcROStestlink/torque distributer for y axis zmp (joint 6)/torque control based on foot in air or on ground/Torque distribute ==
  coeff : Inport
  total torque : Inport  Port=2
  Action Port : ActionPort  ActionType=else
  Gain : Gain
  Product : Product
  torque : Outport
  wires:
  coeff/1 -> Product/1
  total torque/1 -> Product/2
  Product/1 -> Gain/1
  Gain/1 -> torque/1

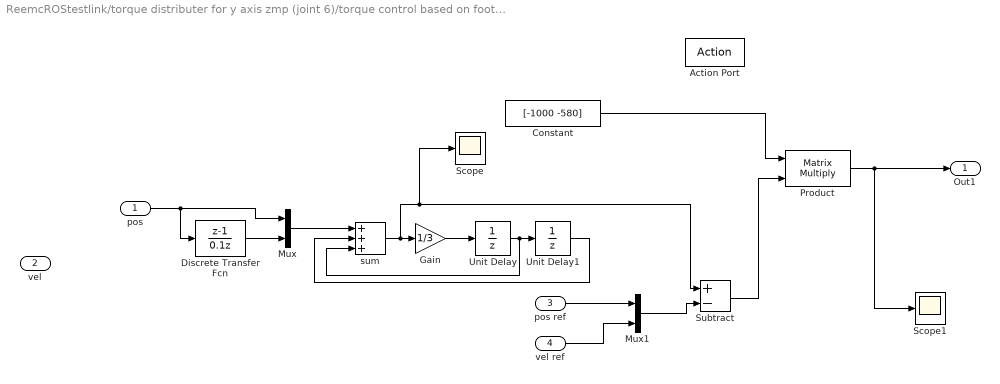
== system ReemcROStestlink/torque distributer for y axis zmp (joint 6)/torque control based on foot in air or on ground/position control ==
  pos : Inport
  vel : Inport  Port=2
  pos ref : Inport  Port=3
  vel ref : Inport  Port=4
  Action Port : ActionPort  ActionType=then
  Constant : Constant  Value=[-1000 -580]  VectorParams1D=off
  Discrete Transfer Fcn : DiscreteTransferFcn  Numerator=[1 -1]  Denominator=[0.1 0]  SampleTime=0.1
  Gain : Gain  Gain=1/3
  Mux : Mux  Inputs=[1;1]
  Mux1 : Mux  Inputs=[1;1]
  Product : Product  Multiplication=Matrix(*)
  Scope : Scope
      settings: YMin=-40  YMax=40  SaveName=ScopeData7
  Scope1 : Scope
      settings: SaveName=ScopeData8
  Subtract : Sum  Inputs=+-
  Unit Delay : UnitDelay  SampleTime=-1
  Unit Delay1 : UnitDelay  SampleTime=-1
  sum : Sum  Inputs=+++
  Out1 : Outport
  wires:
  pos/1 -> Discrete Transfer Fcn/1, Mux/1
  Constant/1 -> Product/1
  Product/1 -> Scope1/1, Out1/1
  vel ref/1 -> Mux1/2
  pos ref/1 -> Mux1/1
  Mux1/1 -> Subtract/2
  Subtract/1 -> Product/2
  Mux/1 -> sum/1
  sum/1 -> Scope/1, Subtract/1, Gain/1
  Gain/1 -> Unit Delay/1
  Unit Delay/1 -> sum/3, Unit Delay1/1
  Unit Delay1/1 -> sum/2
  Discrete Transfer Fcn/1 -> Mux/2

== system ReemcROStestlink/torque distributer for y axis zmp (joint 6)/torque control based on foot in air or on ground 2/Torque distribute ==
  coeff : Inport
  total torque : Inport  Port=2
  Action Port : ActionPort  ActionType=else
  Gain : Gain
  Product : Product
  torque : Outport
  wires:
  coeff/1 -> Product/1
  total torque/1 -> Product/2
  Product/1 -> Gain/1
  Gain/1 -> torque/1

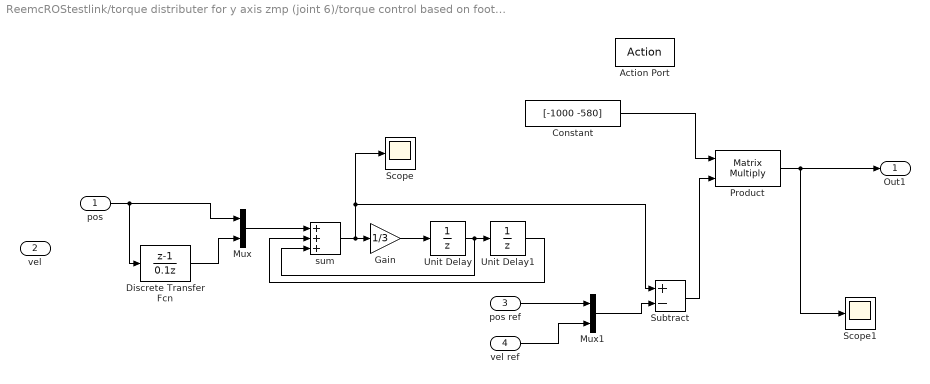
== system ReemcROStestlink/torque distributer for y axis zmp (joint 6)/torque control based on foot in air or on ground 2/position control ==
  pos : Inport
  vel : Inport  Port=2
  pos ref : Inport  Port=3
  vel ref : Inport  Port=4
  Action Port : ActionPort  ActionType=then
  Constant : Constant  Value=[-1000 -580]  VectorParams1D=off
  Discrete Transfer Fcn : DiscreteTransferFcn  Numerator=[1 -1]  Denominator=[0.1 0]  SampleTime=0.1
  Gain : Gain  Gain=1/3
  Mux : Mux  Inputs=[1;1]
  Mux1 : Mux  Inputs=[1;1]
  Product : Product  Multiplication=Matrix(*)
  Scope : Scope
      settings: YMin=-25  YMax=15  SaveName=ScopeData9
  Scope1 : Scope
      settings: YMin=-300  YMax=0  SaveName=ScopeData10
  Subtract : Sum  Inputs=+-
  Unit Delay : UnitDelay  SampleTime=-1
  Unit Delay1 : UnitDelay  SampleTime=-1
  sum : Sum  Inputs=+++
  Out1 : Outport
  wires:
  pos/1 -> Discrete Transfer Fcn/1, Mux/1
  Constant/1 -> Product/1
  Product/1 -> Scope1/1, Out1/1
  vel ref/1 -> Mux1/2
  pos ref/1 -> Mux1/1
  Mux1/1 -> Subtract/2
  Subtract/1 -> Product/2
  Mux/1 -> sum/1
  sum/1 -> Scope/1, Subtract/1, Gain/1
  Gain/1 -> Unit Delay/1
  Unit Delay/1 -> sum/3, Unit Delay1/1
  Unit Delay1/1 -> sum/2
  Discrete Transfer Fcn/1 -> Mux/2

== matlab function ReemcROStestlink/alpha generator from true distances ==
  data: plx input; y output; ply input; prx input; pry input; zmpx input; zmpy input
function y = fcn(plx,ply,prx,pry,zmpx,zmpy)
%#codegen
% plx=position left x, ply position left y etc..

leftDistance=sqrt((zmpx-plx)^2+(zmpy-ply)^2);
rightDistance=sqrt((zmpx-prx)^2+(zmpy-pry)^2);
c=0.03;% the range zmp that is deem to be within a foot

if leftDistance<=c
    a=1;
elseif rightDistance<=c
    a=0;
else
    a=(rightDistance-c)/(leftDistance+rightDistance-2*c);
end
% a=(rightDistanceSquared)/(leftDistanceSquared+rightDistanceSquared);
% 
% if a>0.8
%     a=1;
% elseif a<0.2
%     a=0;
% end

y = a;
